simulink model "SPGF_FSK_0000_R2019b"  (R2019b)
settings: Solver=ode3  SolverName=ode4  StartTime=0.0  StopTime=1.4  FixedStep=50e-6/50  RelTol=1e-3  EnableMultiTasking=on
undefined symbols (not defined in the file): D11, Delta
libraries: powerlib x2544, powerlib_meascontrol x204, simulink x24
(part 20 of 33)

== system SPGF_FSK_0000_R2019b/W32/DPL ==
  Ccs2/1 : powerlib/Elements/Series RLC Branch  LConnTagsString=__new0  RConnTagsString=__new0  BranchType=R  Resistance=-Rg_matrix(3,4)*2  Inductance=1e-3  SetiL0=off  InitialCurrent=0  Capacitance=Rg_matrix(3,4)*2  Setx0=off  InitialVoltage=0  Measurements=None
  Ccs2/3 : powerlib/Elements/Series RLC Branch  LConnTagsString=__new0  RConnTagsString=__new0  BranchType=R  Resistance=-Rg_matrix(3,4)*2  Inductance=1e-3  SetiL0=off  InitialCurrent=0  Capacitance=Rg_matrix(3,4)*2  Setx0=off  InitialVoltage=0  Measurements=None
  Ccs3/1 : powerlib/Elements/Series RLC Branch  LConnTagsString=__new0  RConnTagsString=__new0  BranchType=R  Resistance=-Rg_matrix(5,6)*2  Inductance=1e-3  SetiL0=off  InitialCurrent=0  Capacitance=-C_matrix(5,6)/2  Setx0=off  InitialVoltage=0  Measurements=None
  Ccs3/3 : powerlib/Elements/Series RLC Branch  LConnTagsString=__new0  RConnTagsString=__new0  BranchType=R  Resistance=-Rg_matrix(5,6)*2  Inductance=1e-3  SetiL0=off  InitialCurrent=0  Capacitance=-C_matrix(5,6)/2  Setx0=off  InitialVoltage=0  Measurements=None
  DPL : powerlib/Elements/Distributed Parameters Line  Phases=6  Length=LineLength  Frequency=Frequency  Resistance=R_matrix  Inductance=L_matrix  Capacitance=C_matrix  x1=[-2.15e-05 -1.53014718047574 0 -11.9975076801494 0 0 -9002.7612999088;-2.1e-05 -1.53058650120651 0 -12.0009749818967 0 0 -9001.97102364387;-2.05e-05 -1.53102578417156 0 -12.0044419875317 0 0 -9001.18052526422;-2e-05 -1.53146502936007 0 -12.0079086969691 0 0 -9000.38980478933;-1.95e-05 -1.5319042367612 0 -12.0113751101231 0 0 -8999.59886223873;-1.9e-05 -1.5323434063641 0 -12.0148412269084 0 0 -8998.80769763193;-1.85e-05 -1.53278253815794 0 -12.0183070472393 0 0 -8998.01631098845;-1.8e-05 -1.53322163213189 0 -12.0217725710304 0 0 -8997.22470232782;-1.75e-05 -1.53366068827512 0 -12.0252377981962 0 0 -8996.43287166957;-1.7e-05 -1.53409970657678 0 -12.0287027286511 0 0 -8995.64081903323;-1.65e-05 -1.53453868702605 0 -12.0321673623096 0 0 -8994.84854443835;-1.6e-05 -1.5349776296121 0 -12.0356316990864 0 0 -8994.05604790448;-1.55e-05 -1.53541653432409 0 -12.0390957388958 0 0 -8993.26332945117;-1.5e-05 -1.53585540115119 0 -12.0425594816524 0 0 -8992.47038909799;-1.45e-05 -1.53629423008259 0 -12.0460229272708 0 0 -8991.67722686449;-1.4e-05 -1.53673302110744 0 -12.0494860756655 0 0 -8990.88384277025;-1.35e-05 -1.53717177421492 0 -12.052948926751 0 0 -8990.09023683485;-1.3e-05 -1.53761048939422 0 -12.056411480442 0 0 -8989.29640907786;-1.25e-05 -1.53804916663449 0 -12.0598737366529 0 0 -8988.50235951887;-1.2e-05 -1.53848780592492 0 -12.0633356952984 0 0 -8987.70808817747;-1.15e-05 -1.53892640725469 0 -12.066797356293 0 0 -8986.91359507327;-1.1e-05 -1.53936497061297 0 -12.0702587195513 0 0 -8986.11888022586;-1.05e-05 -1.53980349598894 0 -12.0737197849879 0 0 -8985.32394365486;-1e-05 -1.54024198337178 0 -12.0771805525174 0 0 -8984.52878537988;-9.5e-06 -1.54068043275068 0 -12.0806410220544 0 0 -8983.73340542053;-9e-06 -1.54111884411481 0 -12.0841011935135 0 0 -8982.93780379645;-8.5e-06 -1.54155721745336 0 -12.0875610668094 0 0 -8982.14198052726;-8e-06 -1.5419955527555 0 -12.0910206418567 0 0 -8981.3459356326;-7.5e-06 -1.54243385001044 0 -12.09447991857 0 0 -8980.54966913212;-7e-06 -1.54287210920734 0 -12.097938896864 0 0 -8979.75318104545;-6.5e-06 -1.5433103303354 0 -12.1013975766533 0 0 -8978.95647139226;-6e-06 -1.5437485133838 0 -12.1048559578526 0 0 -8978.15954019219;-5.5e-06 -1.54418665834174 0 -12.1083140403766 0 0 -8977.36238746492;-5e-06 -1.54462476519839 0 -12.1117718241398 0 0 -8976.56501323011;-4.5e-06 -1.54506283394296 0 -12.1152293090571 0 0 -8975.76741750744;-4e-06 -1.54550086456463 0 -12.1186864950431 -2674.88891077229 0 -8974.96960031658;-3.5e-06 -1.5459388570526 5072.52279858498 -12.1221433820125 -2675.63246615166 4735.28985862403 -8974.17156167723;-3e-06 -1.54637681139605 5073.93232204557 -12.12559996988 -2676.37595551245 4734.86865062958 -8973.37330160906;-2.5e-06 -1.54681472758419 5075.3417203119 -12.1290562585602 -2677.1193788363 4734.44732580693 -8972.57482013179;-2e-06 -1.5472526056062 5076.75099334919 -12.1325122479681 -2677.86273610488 4734.02588416648 -8971.77611726511;-1.5e-06 -1.54769044545128 5078.16014112268 -12.1359679380182 -2678.60602729985 4733.60432571862 -8970.97719302872;-1e-06 -1.54812824710863 5079.56916359758 -12.1394233286252 -2679.34925240286 4733.18265047376 -8970.17804744235;-5e-07 -1.54856601056745 5080.97806073914 -12.1428784197041 -2680.09241139558 4732.76085844229 -8969.3786805257]  x2=[-2.15e-05 -1.52937369923623 0 -11.9860465797701 0 0 -9022.25103677801;-2.1e-05 -1.52981566216544 0 -11.9895391205462 0 0 -9021.46040632605;-2.05e-05 -1.53025758734796 0 -11.9930313654924 0 0 -9020.66955327848;-2e-05 -1.5306994747729 0 -11.9965233145224 0 0 -9019.87847765481;-1.95e-05 -1.53114132442933 0 -12.00001496755 0 0 -9019.08717947456;-1.9e-05 -1.53158313630637 0 -12.0035063244892 0 0 -9018.29565875726;-1.85e-05 -1.53202491039311 0 -12.0069973852536 0 0 -9017.50391552242;-1.8e-05 -1.53246664667865 0 -12.0104881497573 0 0 -9016.7119497896;-1.75e-05 -1.53290834515209 0 -12.0139786179141 0 0 -9015.91976157833;-1.7e-05 -1.53335000580254 0 -12.0174687896379 0 0 -9015.12735090815;-1.65e-05 -1.53379162861909 0 -12.0209586648425 0 0 -9014.33471779863;-1.6e-05 -1.53423321359085 0 -12.0244482434418 0 0 -9013.54186226931;-1.55e-05 -1.53467476070692 0 -12.0279375253497 0 0 -9012.74878433976;-1.5e-05 -1.5351162699564 0 -12.0314265104802 0 0 -9011.95548402955;-1.45e-05 -1.53555774132842 0 -12.0349151987472 0 0 -9011.16196135825;-1.4e-05 -1.53599917481206 0 -12.0384035900645 0 0 -9010.36821634544;-1.35e-05 -1.53644057039645 0 -12.0418916843461 0 0 -9009.57424901071;-1.3e-05 -1.53688192807068 0 -12.0453794815059 0 0 -9008.78005937364;-1.25e-05 -1.53732324782387 0 -12.0488669814579 0 0 -9007.98564745383;-1.2e-05 -1.53776452964513 0 -12.0523541841161 0 0 -9007.19101327089;-1.15e-05 -1.53820577352357 0 -12.0558410893943 0 0 -9006.39615684442;-1.1e-05 -1.53864697944831 0 -12.0593276972066 0 0 -9005.60107819403;-1.05e-05 -1.53908814740845 0 -12.0628140074669 0 0 -9004.80577733934;-1e-05 -1.53952927739312 0 -12.0663000200891 0 0 -9004.01025429998;-9.5e-06 -1.53997036939142 0 -12.0697857349874 0 0 -9003.21450909557;-9e-06 -1.54041142339248 0 -12.0732711520756 0 0 -9002.41854174574;-8.5e-06 -1.54085243938541 0 -12.0767562712678 0 0 -9001.62235227014;-8e-06 -1.54129341735933 0 -12.080241092478 0 0 -9000.82594068841;-7.5e-06 -1.54173435730336 0 -12.0837256156202 0 0 -9000.02930702021;-7e-06 -1.54217525920661 0 -12.0872098406084 0 0 -8999.23245128518;-6.5e-06 -1.54261612305822 0 -12.0906937673567 0 0 -8998.43537350299;-6e-06 -1.5430569488473 0 -12.0941773957791 0 0 -8997.63807369331;-5.5e-06 -1.54349773656298 0 -12.0976607257895 0 0 -8996.84055187581;-5e-06 -1.54393848619438 0 -12.1011437573022 0 0 -8996.04280807017;-4.5e-06 -1.54437919773062 0 -12.1046264902311 0 0 -8995.24484229607;-4e-06 -1.54481987116083 0 -12.1081089244904 -2677.09103389761 0 -8994.4466545732;-3.5e-06 -1.54526050647415 5076.70076594894 -12.111591059994 -2677.83624236647 4745.56687862651 -8993.64824492125;-3e-06 -1.54570110365968 5078.11342326981 -12.1150728966561 -2678.58138476238 4745.14547461087 -8992.84961335993;-2.5e-06 -1.54614166270657 5079.52595529325 -12.1185544343908 -2679.32646106693 4744.72395351346 -8992.05075990894;-2e-06 -1.54658218360395 5080.93836198442 -12.1220356731121 -2680.07147126176 4744.30231534468 -8991.25168458799;-1.5e-06 -1.54702266634093 5082.35064330845 -12.1255166127341 -2680.81641532848 4743.88056011494 -8990.45238741679;-1e-06 -1.54746311090667 5083.76279923051 -12.1289972531711 -2681.5612932487 4743.45868783463 -8989.65286841508;-5e-07 -1.54790351729028 5085.17482971575 -12.132477594337 -2682.30610500404 4743.03669851417 -8988.85312760257]  x3=[-2.15e-05 0.00477826196837518 0 -0.618760489523996 0 0 -226.302645481419;-2.1e-05 0.00477462202162191 0 -0.619060199625067 0 0 -226.29417562915;-2.05e-05 0.00477098195705956 0 -0.619359894451439 0 0 -226.285700193296;-2e-05 0.00476734177477795 0 -0.619659573995719 0 0 -226.277219174067;-1.95e-05 0.00476370147486689 0 -0.619959238250512 0 0 -226.26873257167;-1.9e-05 0.00476006105741622 0 -0.620258887208423 0 0 -226.260240386317;-1.85e-05 0.00475642052251574 0 -0.62055852086206 0 0 -226.251742618216;-1.8e-05 0.00475277987025529 0 -0.620858139204029 0 0 -226.243239267577;-1.75e-05 0.0047491391007247 0 -0.621157742226938 0 0 -226.234730334609;-1.7e-05 0.0047454982140138 0 -0.621457329923394 0 0 -226.226215819524;-1.65e-05 0.00474185721021243 0 -0.621756902286004 0 0 -226.21769572253;-1.6e-05 0.00473821608941042 0 -0.622056459307379 0 0 -226.209170043839;-1.55e-05 0.00473457485169761 0 -0.622356000980125 0 0 -226.20063878366;-1.5e-05 0.00473093349716385 0 -0.622655527296852 0 0 -226.192101942204;-1.45e-05 0.00472729202589899 0 -0.622955038250171 0 0 -226.183559519681;-1.4e-05 0.00472365043799287 0 -0.623254533832689 0 0 -226.175011516303;-1.35e-05 0.00472000873353535 0 -0.623554014037019 0 0 -226.16645793228;-1.3e-05 0.00471636691261628 0 -0.62385347885577 0 0 -226.157898767824;-1.25e-05 0.00471272497532552 0 -0.624152928281553 0 0 -226.149334023145;-1.2e-05 0.00470908292175294 0 -0.62445236230698 0 0 -226.140763698455;-1.15e-05 0.00470544075198839 0 -0.624751780924663 0 0 -226.132187793965;-1.1e-05 0.00470179846612174 0 -0.625051184127214 0 0 -226.123606309887;-1.05e-05 0.00469815606424287 0 -0.625350571907245 0 0 -226.115019246433;-1e-05 0.00469451354644164 0 -0.625649944257368 0 0 -226.106426603814;-9.5e-06 0.00469087091280794 0 -0.625949301170199 0 0 -226.097828382243;-9e-06 0.00468722816343163 0 -0.626248642638349 0 0 -226.089224581932;-8.5e-06 0.00468358529840261 0 -0.626547968654434 0 0 -226.080615203092;-8e-06 0.00467994231781075 0 -0.626847279211067 0 0 -226.072000245937;-7.5e-06 0.00467629922174594 0 -0.627146574300863 0 0 -226.063379710679;-7e-06 0.00467265601029807 0 -0.627445853916438 0 0 -226.054753597531;-6.5e-06 0.00466901268355704 0 -0.627745118050407 0 0 -226.046121906705;-6e-06 0.00466536924161274 0 -0.628044366695387 0 0 -226.037484638415;-5.5e-06 0.00466172568455507 0 -0.628343599843992 0 0 -226.028841792873;-5e-06 0.00465808201247392 0 -0.628642817488841 0 0 -226.020193370294;-4.5e-06 0.00465443822545921 0 -0.62894201962255 0 0 -226.011539370889;-4e-06 0.00465079432360084 0 -0.629241206237737 -222.82339661273 0 -226.002879794873;-3.5e-06 0.00464715030698872 42.9134986181816 -0.629540377327019 -222.889214995494 448.335934563766 -225.99421464246;-3e-06 0.00464350617571277 42.9459643816412 -0.629839532883015 -222.955027878687 448.298611391661 -225.985543913863;-2.5e-06 0.00463986192986288 42.9784290854516 -0.630138672898344 -223.020835260686 448.261277158231 -225.976867609297;-2e-06 0.004636217569529 43.0108927288118 -0.630437797365624 -223.086637139865 448.223931864398 -225.968185728974;-1.5e-06 0.00463257309480103 43.0433553109208 -0.630736906277475 -223.152433514603 448.186575511082 -225.95949827311;-1e-06 0.00462892850576891 43.0758168309775 -0.631035999626517 -223.218224383275 448.149208099206 -225.950805241919;-5e-07 0.00462528380252255 43.1082772881811 -0.631335077405369 -223.284009744258 448.111829629691 -225.942106635616]  x4=[-2.15e-05 -0.0246566983072682 0 -0.809678743743674 0 0 -37.8270818179801;-2.1e-05 -0.0246588297990929 0 -0.809794272225366 0 0 -37.8124114690117;-2.05e-05 -0.0246609606824854 0 -0.809909780726186 0 0 -37.7977401870595;-2e-05 -0.0246630909573931 0 -0.810025269243283 0 0 -37.7830679724853;-1.95e-05 -0.0246652206237634 0 -0.810140737773807 0 0 -37.7683948256514;-1.9e-05 -0.0246673496815438 0 -0.81025618631491 0 0 -37.7537207469197;-1.85e-05 -0.0246694781306817 0 -0.810371614863743 0 0 -37.7390457366522;-1.8e-05 -0.0246716059711247 0 -0.810487023417458 0 0 -37.7243697952112;-1.75e-05 -0.0246737332028202 0 -0.810602411973208 0 0 -37.7096929229586;-1.7e-05 -0.0246758598257157 0 -0.810717780528144 0 0 -37.6950151202566;-1.65e-05 -0.0246779858397588 0 -0.810833129079422 0 0 -37.6803363874674;-1.6e-05 -0.024680111244897 0 -0.810948457624193 0 0 -37.6656567249532;-1.55e-05 -0.0246822360410779 0 -0.811063766159614 0 0 -37.6509761330762;-1.5e-05 -0.024684360228249 0 -0.811179054682838 0 0 -37.6362946121986;-1.45e-05 -0.0246864838063579 0 -0.811294323191021 0 0 -37.6216121626826;-1.4e-05 -0.0246886067753522 0 -0.81140957168132 0 0 -37.6069287848905;-1.35e-05 -0.0246907291351796 0 -0.811524800150889 0 0 -37.5922444791847;-1.3e-05 -0.0246928508857877 0 -0.811640008596887 0 0 -37.5775592459274;-1.25e-05 -0.0246949720271241 0 -0.811755197016471 0 0 -37.562873085481;-1.2e-05 -0.0246970925591365 0 -0.811870365406797 0 0 -37.5481859982079;-1.15e-05 -0.0246992124817726 0 -0.811985513765026 0 0 -37.5334979844704;-1.1e-05 -0.02470133179498 0 -0.812100642088315 0 0 -37.518809044631;-1.05e-05 -0.0247034504987065 0 -0.812215750373824 0 0 -37.5041191790521;-1e-05 -0.0247055685928998 0 -0.812330838618713 0 0 -37.4894283880961;-9.5e-06 -0.0247076860775076 0 -0.812445906820141 0 0 -37.4747366721256;-9e-06 -0.0247098029524777 0 -0.81256095497527 0 0 -37.460044031503;-8.5e-06 -0.0247119192177578 0 -0.812675983081262 0 0 -37.4453504665908;-8e-06 -0.0247140348732958 0 -0.812790991135277 0 0 -37.4306559777517;-7.5e-06 -0.0247161499190394 0 -0.812905979134479 0 0 -37.4159605653482;-7e-06 -0.0247182643549365 0 -0.813020947076029 0 0 -37.4012642297428;-6.5e-06 -0.0247203781809348 0 -0.813135894957092 0 0 -37.3865669712983;-6e-06 -0.0247224913969823 0 -0.813250822774831 0 0 -37.3718687903771;-5.5e-06 -0.0247246040030267 0 -0.81336573052641 0 0 -37.3571696873421;-5e-06 -0.024726715999016 0 -0.813480618208994 0 0 -37.3424696625559;-4.5e-06 -0.024728827384898 0 -0.813595485819749 0 0 -37.3277687163811;-4e-06 -0.0247309381606206 0 -0.813710333355839 -211.777509166727 0 -37.3130668491806;-3.5e-06 -0.0247330483261319 84.5050032625513 -0.813825160814432 -211.832740480619 382.91660687957 -37.2983640613171;-3e-06 -0.0247351578813796 84.5080140470438 -0.813939968192694 -211.887966567748 382.880140777377 -37.2836603531533;-2.5e-06 -0.0247372668263117 84.5110227463845 -0.814054755487792 -211.943187426751 382.843665227995 -37.268955725052;-2e-06 -0.0247393751608763 84.5140293604994 -0.814169522696895 -211.998403056265 382.807180232325 -37.2542501773762;-1.5e-06 -0.0247414828850213 84.5170338893141 -0.814284269817169 -212.053613454928 382.770685791266 -37.2395437104886;-1e-06 -0.0247435899986946 84.5200363327547 -0.814398996845785 -212.108818621378 382.734181905718 -37.224836324752;-5e-07 -0.0247456965018443 84.5230366907469 -0.814513703779911 -212.164018554253 382.697668576584 -37.2101280205295]  x5=2.11324941411031e-05  V1=ones(3,3)  V2=ones(3,3)  I1=ones(3,3)  I2=ones(3,3)  nHarmo=1  Measurements=None  Decoupling=off  VsMag0=0  VrMag0=0  VsAngle0=0  VrAngle0=0  IsMag0=0  IrMag0=0  IsAngle0=0  IrAngle0=0
  Ground{1..4} (4 alike) : powerlib/Elements/Ground  LConnTagsString=a
  Rcs*1 : powerlib/Elements/Series RLC Branch  LConnTagsString=__new0  RConnTagsString=__new0  BranchType=R  Resistance=-Rg_matrix(1,2)*2  Inductance=1e-3  SetiL0=off  InitialCurrent=0  Capacitance=Rg_matrix(1,2)*2  Setx0=off  InitialVoltage=0  Measurements=None
  Rcs*2 : powerlib/Elements/Series RLC Branch  LConnTagsString=__new0  RConnTagsString=__new0  BranchType=R  Resistance=-Rg_matrix(1,2)*2  Inductance=1e-3  SetiL0=off  InitialCurrent=0  Capacitance=Rg_matrix(1,2)*2  Setx0=off  InitialVoltage=0  Measurements=None
  Rgsg1/1 : powerlib/Elements/Series RLC Branch  LConnTagsString=__new0  RConnTagsString=__new0  BranchType=R  Resistance=(Rg_matrix(4,4)+Rg_matrix(3,4))*2  Inductance=1e-3  SetiL0=off  InitialCurrent=0  Capacitance=Rg_matrix(1,2)*2  Setx0=off  InitialVoltage=0  Measurements=None
  Rgsg1/2 : powerlib/Elements/Series RLC Branch  LConnTagsString=__new0  RConnTagsString=__new0  BranchType=R  Resistance=(Rg_matrix(2,2)+Rg_matrix(1,2))*2  Inductance=1e-3  SetiL0=off  InitialCurrent=0  Capacitance=Rg_matrix(1,2)*2  Setx0=off  InitialVoltage=0  Measurements=None
  Rgsg1/3 : powerlib/Elements/Series RLC Branch  LConnTagsString=__new0  RConnTagsString=__new0  BranchType=R  Resistance=(Rg_matrix(4,4)+Rg_matrix(3,4))*2  Inductance=1e-3  SetiL0=off  InitialCurrent=0  Capacitance=Rg_matrix(1,2)*2  Setx0=off  InitialVoltage=0  Measurements=None
  Rgsg1/4 : powerlib/Elements/Series RLC Branch  LConnTagsString=__new0  RConnTagsString=__new0  BranchType=R  Resistance=(Rg_matrix(2,2)+Rg_matrix(1,2))*2  Inductance=1e-3  SetiL0=off  InitialCurrent=0  Capacitance=Rg_matrix(1,2)*2  Setx0=off  InitialVoltage=0  Measurements=None
  Rsg*1 : powerlib/Elements/Series RLC Branch  LConnTagsString=__new0  RConnTagsString=__new0  BranchType=R  Resistance=(Rg_matrix(6,6)+Rg_matrix(5,6))*2  Inductance=1e-3  SetiL0=off  InitialCurrent=0  Capacitance=Rg_matrix(1,2)*2  Setx0=off  InitialVoltage=0  Measurements=None
  Rsg*2 : powerlib/Elements/Series RLC Branch  LConnTagsString=__new0  RConnTagsString=__new0  BranchType=R  Resistance=(Rg_matrix(6,6)+Rg_matrix(5,6))*2  Inductance=1e-3  SetiL0=off  InitialCurrent=0  Capacitance=Rg_matrix(1,2)*2  Setx0=off  InitialVoltage=0  Measurements=None
  A : PMIOPort  Side=Left
  B : PMIOPort  Port=2  Side=Left
  C : PMIOPort  Port=3  Side=Left
  a : PMIOPort  Port=4  Side=Right
  b : PMIOPort  Port=5  Side=Right
  c : PMIOPort  Port=6  Side=Right
  connections:
  c/RConn1 -- Ccs3/1/RConn1 -- DPL/RConn5
  b/RConn1 -- Ccs2/1/RConn1 -- DPL/RConn3
  a/RConn1 -- DPL/RConn1 -- Rcs*1/RConn1
  Ground4/LConn1 -- DPL/RConn6 -- Ccs3/1/LConn1 -- Rsg*1/LConn1 -- Rcs*1/LConn1 -- Rgsg1/4/LConn1 -- DPL/RConn2 -- DPL/RConn4 -- Ccs2/1/LConn1 -- Rgsg1/3/LConn1
  Ground1/LConn1 -- Rgsg1/4/RConn1 -- Rsg*1/RConn1 -- Rgsg1/3/RConn1
  Ground3/LConn1 -- Ccs3/3/LConn1 -- Rsg*2/LConn1 -- DPL/LConn6 -- Rgsg1/1/LConn1 -- Ccs2/3/LConn1 -- DPL/LConn4 -- Rgsg1/2/LConn1 -- Rcs*2/LConn1 -- DPL/LConn2
  Ground2/LConn1 -- Rgsg1/1/RConn1 -- Rsg*2/RConn1 -- Rgsg1/2/RConn1
  Ccs3/3/RConn1 -- DPL/LConn5 -- C/RConn1
  Ccs2/3/RConn1 -- DPL/LConn3 -- B/RConn1
  Rcs*2/RConn1 -- DPL/LConn1 -- A/RConn1

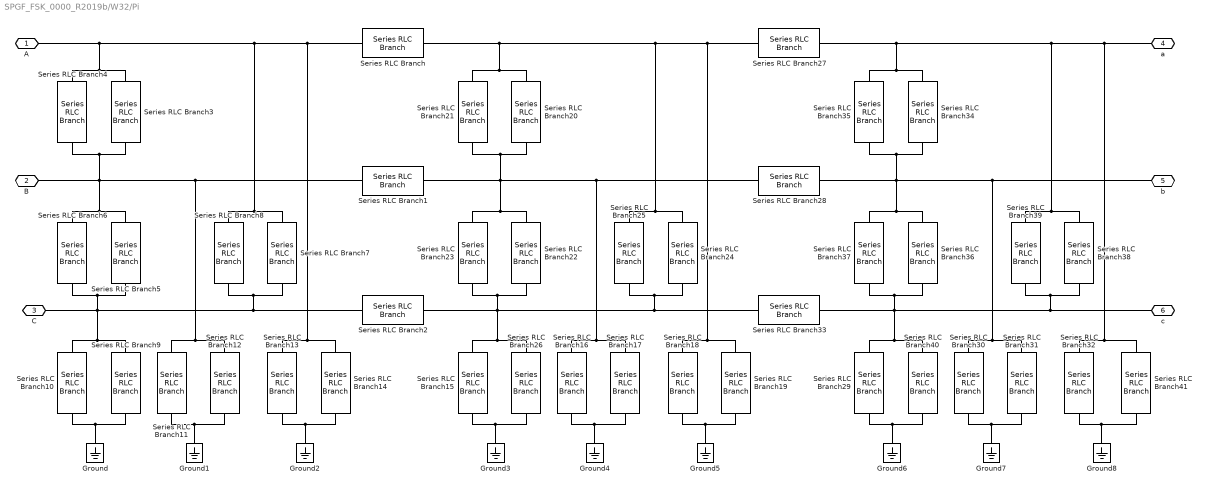
== system SPGF_FSK_0000_R2019b/W32/Pi ==
  Ground{,1..8} (9 alike) : powerlib/Elements/Ground  LConnTagsString=a
  Series RLC Branch{,1..2,27..28,33} (6 alike) : powerlib/Elements/Series RLC Branch  LConnTagsString=__new0  RConnTagsString=__new0  BranchType=RL  Resistance=R/2  Inductance=L/2  SetiL0=off  InitialCurrent=0  Capacitance=1e-6  Setx0=off  InitialVoltage=0  Measurements=None
  Series RLC Branch{10..11,13,29..30,32} (6 alike) : powerlib/Elements/Series RLC Branch  LConnTagsString=__new0  RConnTagsString=__new0  BranchType=R  Resistance=Rfg*4  Inductance=L/2  SetiL0=off  InitialCurrent=0  Capacitance=1e-6  Setx0=off  InitialVoltage=0  Measurements=None
  Series RLC Branch{9,12,14,31,40..41} (6 alike) : powerlib/Elements/Series RLC Branch  LConnTagsString=__new0  RConnTagsString=__new0  BranchType=C  Resistance=R/2  Inductance=L/2  SetiL0=off  InitialCurrent=0  Capacitance=Cfg*0.25  Setx0=off  InitialVoltage=0  Measurements=None
  Series RLC Branch15 : powerlib/Elements/Series RLC Branch  LConnTagsString=__new0  RConnTagsString=__new0  BranchType=R  Resistance=Rfg*2  Inductance=L/2  SetiL0=off  InitialCurrent=0  Capacitance=1e-6  Setx0=off  InitialVoltage=0  Measurements=None
  Series RLC Branch16 : powerlib/Elements/Series RLC Branch  LConnTagsString=__new0  RConnTagsString=__new0  BranchType=R  Resistance=Rfg*2  Inductance=L/2  SetiL0=off  InitialCurrent=0  Capacitance=1e-6  Setx0=off  InitialVoltage=0  Measurements=None
  Series RLC Branch17 : powerlib/Elements/Series RLC Branch  LConnTagsString=__new0  RConnTagsString=__new0  BranchType=C  Resistance=R/2  Inductance=L/2  SetiL0=off  InitialCurrent=0  Capacitance=Cfg*0.5  Setx0=off  InitialVoltage=0  Measurements=None
  Series RLC Branch18 : powerlib/Elements/Series RLC Branch  LConnTagsString=__new0  RConnTagsString=__new0  BranchType=R  Resistance=Rfg*2  Inductance=L/2  SetiL0=off  InitialCurrent=0  Capacitance=1e-6  Setx0=off  InitialVoltage=0  Measurements=None
  Series RLC Branch19 : powerlib/Elements/Series RLC Branch  LConnTagsString=__new0  RConnTagsString=__new0  BranchType=C  Resistance=R/2  Inductance=L/2  SetiL0=off  InitialCurrent=0  Capacitance=Cfg*0.5  Setx0=off  InitialVoltage=0  Measurements=None
  Series RLC Branch20 : powerlib/Elements/Series RLC Branch  LConnTagsString=__new0  RConnTagsString=__new0  BranchType=C  Resistance=R/2  Inductance=L/2  SetiL0=off  InitialCurrent=0  Capacitance=Cmf*0.5  Setx0=off  InitialVoltage=0  Measurements=None
  Series RLC Branch21 : powerlib/Elements/Series RLC Branch  LConnTagsString=__new0  RConnTagsString=__new0  BranchType=R  Resistance=Rmf*2  Inductance=L/2  SetiL0=off  InitialCurrent=0  Capacitance=1e-6  Setx0=off  InitialVoltage=0  Measurements=None
  Series RLC Branch22 : powerlib/Elements/Series RLC Branch  LConnTagsString=__new0  RConnTagsString=__new0  BranchType=C  Resistance=R/2  Inductance=L/2  SetiL0=off  InitialCurrent=0  Capacitance=Cmf*0.5  Setx0=off  InitialVoltage=0  Measurements=None
  Series RLC Branch23 : powerlib/Elements/Series RLC Branch  LConnTagsString=__new0  RConnTagsString=__new0  BranchType=R  Resistance=Rmf*2  Inductance=L/2  SetiL0=off  InitialCurrent=0  Capacitance=1e-6  Setx0=off  InitialVoltage=0  Measurements=None
  Series RLC Branch24 : powerlib/Elements/Series RLC Branch  LConnTagsString=__new0  RConnTagsString=__new0  BranchType=C  Resistance=R/2  Inductance=L/2  SetiL0=off  InitialCurrent=0  Capacitance=Cmf*0.5  Setx0=off  InitialVoltage=0  Measurements=None
  Series RLC Branch25 : powerlib/Elements/Series RLC Branch  LConnTagsString=__new0  RConnTagsString=__new0  BranchType=R  Resistance=Rmf*2  Inductance=L/2  SetiL0=off  InitialCurrent=0  Capacitance=1e-6  Setx0=off  InitialVoltage=0  Measurements=None
  Series RLC Branch26 : powerlib/Elements/Series RLC Branch  LConnTagsString=__new0  RConnTagsString=__new0  BranchType=C  Resistance=R/2  Inductance=L/2  SetiL0=off  InitialCurrent=0  Capacitance=Cfg*0.5  Setx0=off  InitialVoltage=0  Measurements=None
  Series RLC Branch{3,5,7,34,36,38} (6 alike) : powerlib/Elements/Series RLC Branch  LConnTagsString=__new0  RConnTagsString=__new0  BranchType=C  Resistance=R/2  Inductance=L/2  SetiL0=off  InitialCurrent=0  Capacitance=Cmf*0.25  Setx0=off  InitialVoltage=0  Measurements=None
  Series RLC Branch{4,6,8,35,37,39} (6 alike) : powerlib/Elements/Series RLC Branch  LConnTagsString=__new0  RConnTagsString=__new0  BranchType=R  Resistance=Rmf*4  Inductance=L/2  SetiL0=off  InitialCurrent=0  Capacitance=1e-6  Setx0=off  InitialVoltage=0  Measurements=None
  A : PMIOPort  Side=Left
  B : PMIOPort  Port=2  Side=Left
  C : PMIOPort  Port=3  Side=Left
  a : PMIOPort  Port=4  Side=Right
  b : PMIOPort  Port=5  Side=Right
  c : PMIOPort  Port=6  Side=Right
  connections:
  Ground8/LConn1 -- Series RLC Branch41/RConn1 -- Series RLC Branch32/RConn1
  Ground7/LConn1 -- Series RLC Branch30/RConn1 -- Series RLC Branch31/RConn1
  Ground6/LConn1 -- Series RLC Branch40/RConn1 -- Series RLC Branch29/RConn1
  Series RLC Branch40/LConn1 -- Series RLC Branch33/RConn1 -- Series RLC Branch38/RConn1 -- Series RLC Branch39/RConn1 -- c/RConn1 -- Series RLC Branch37/RConn1 -- Series RLC Branch36/RConn1 -- Series RLC Branch29/LConn1
  Series RLC Branch35/LConn1 -- Series RLC Branch27/RConn1 -- Series RLC Branch39/LConn1 -- Series RLC Branch38/LConn1 -- Series RLC Branch32/LConn1 -- Series RLC Branch41/LConn1 -- a/RConn1 -- Series RLC Branch34/LConn1
  Series RLC Branch30/LConn1 -- Series RLC Branch28/RConn1 -- Series RLC Branch37/LConn1 -- Series RLC Branch36/LConn1 -- Series RLC Branch34/RConn1 -- Series RLC Branch35/RConn1 -- b/RConn1 -- Series RLC Branch31/LConn1
  Series RLC Branch19/RConn1 -- Series RLC Branch18/RConn1 -- Ground5/LConn1
  Series RLC Branch16/RConn1 -- Series RLC Branch17/RConn1 -- Ground4/LConn1
  Ground3/LConn1 -- Series RLC Branch15/RConn1 -- Series RLC Branch26/RConn1
  Series RLC Branch23/RConn1 -- Series RLC Branch22/RConn1 -- Series RLC Branch24/RConn1 -- Series RLC Branch25/RConn1 -- Series RLC Branch33/LConn1 -- Series RLC Branch2/RConn1 -- Series RLC Branch15/LConn1 -- Series RLC Branch26/LConn1
  Series RLC Branch25/LConn1 -- Series RLC Branch24/LConn1 -- Series RLC Branch18/LConn1 -- Series RLC Branch19/LConn1 -- Series RLC Branch27/LConn1 -- Series RLC Branch/RConn1 -- Series RLC Branch20/LConn1 -- Series RLC Branch21/LConn1
  Series RLC Branch21/RConn1 -- Series RLC Branch20/RConn1 -- Series RLC Branch22/LConn1 -- Series RLC Branch23/LConn1 -- Series RLC Branch1/RConn1 -- Series RLC Branch28/LConn1 -- Series RLC Branch16/LConn1 -- Series RLC Branch17/LConn1
  Ground2/LConn1 -- Series RLC Branch14/RConn1 -- Series RLC Branch13/RConn1
  Ground1/LConn1 -- Series RLC Branch11/RConn1 -- Series RLC Branch12/RConn1
  Series RLC Branch10/RConn1 -- Ground/LConn1 -- Series RLC Branch9/RConn1
  Series RLC Branch10/LConn1 -- Series RLC Branch6/RConn1 -- Series RLC Branch5/RConn1 -- C/RConn1 -- Series RLC Branch7/RConn1 -- Series RLC Branch8/RConn1 -- Series RLC Branch2/LConn1 -- Series RLC Branch9/LConn1
  Series RLC Branch14/LConn1 -- Series RLC Branch/LConn1 -- Series RLC Branch8/LConn1 -- Series RLC Branch7/LConn1 -- Series RLC Branch3/LConn1 -- Series RLC Branch4/LConn1 -- A/RConn1 -- Series RLC Branch13/LConn1
  Series RLC Branch1/LConn1 -- Series RLC Branch3/RConn1 -- Series RLC Branch4/RConn1 -- B/RConn1 -- Series RLC Branch6/LConn1 -- Series RLC Branch5/LConn1 -- Series RLC Branch11/LConn1 -- Series RLC Branch12/LConn1

== system SPGF_FSK_0000_R2019b/W32/Q ==
  breaker : Subsystem  Commented=on  mask{SwitchA=off, SwitchB=off, SwitchC=off, InitialStatus=[1 1 1], BreakerResistance=0.0001, SnubberResistance=1e6, SnubberCapacitance=inf, TransitionTimes=[0.5 0.7], ShiftTimes=[0 0 0]}
      mask prompts: SwitchA "Switching of phase A"; SwitchB "Switching of phase B"; SwitchC "Switching of phase C"; InitialStatus "Initial status of phase breaker [A, B, C]"; BreakerResistance "Breaker resistance Ron (ohms) :"; SnubberResistance "Snubbers resistance Rp (ohms) :"; SnubberCapacitance "Snubbers capacitance Cp (F) :"; TransitionTimes "Transition times (s) :"; ShiftTimes "Time differences for switch [tA, tB, tC] (s) :"
      mask init: same as SPGF_FSK_0000_R2019b/Feed/Q/breaker
      mask Display:
      | % port_label('input',1,'Iabc');
      | 
      | port_label('lconn',1,'A');
      | port_label('lconn',2,'B');
      | port_label('lconn',3,'C');
      | 
      | port_label('rconn',1,'a');
      | port_label('rconn',2,'b');
      | port_label('rconn',3,'c');
      | 
      | disp('   Q    ');
  meas : Subsystem
  shunt : Subsystem
  A : PMIOPort  Side=Right
  B : PMIOPort  Port=2  Side=Right
  C : PMIOPort  Port=3  Side=Right
  a : PMIOPort  Port=4  Side=Left
  b : PMIOPort  Port=5  Side=Left
  c : PMIOPort  Port=6  Side=Left
  connections:
  shunt/LConn3 -- C/RConn1 -- breaker/LConn3
  shunt/LConn2 -- B/RConn1 -- breaker/LConn2
  A/RConn1 -- shunt/LConn1 -- breaker/LConn1
  meas/RConn1 -- a/RConn1
  meas/RConn2 -- b/RConn1
  meas/RConn3 -- c/RConn1
  meas/LConn3 -- breaker/RConn3 -- shunt/RConn3
  meas/LConn2 -- breaker/RConn2 -- shunt/RConn2
  meas/LConn1 -- breaker/RConn1 -- shunt/RConn1

== system SPGF_FSK_0000_R2019b/W32/concentrated ==
  Ccs/1 : powerlib/Elements/Series RLC Branch  LConnTagsString=__new0  RConnTagsString=__new0  BranchType=C  Resistance=190  Inductance=1e-3  SetiL0=off  InitialCurrent=0  Capacitance=-C_matrix(1,2)/2  Setx0=off  InitialVoltage=0  Measurements=None
  Ccs/2 : powerlib/Elements/Series RLC Branch  LConnTagsString=__new0  RConnTagsString=__new0  BranchType=C  Resistance=190  Inductance=1e-3  SetiL0=off  InitialCurrent=0  Capacitance=-C_matrix(1,2)/2  Setx0=off  InitialVoltage=0  Measurements=None
  Ccs2/1 : powerlib/Elements/Series RLC Branch  LConnTagsString=__new0  RConnTagsString=__new0  BranchType=C  Resistance=190  Inductance=1e-3  SetiL0=off  InitialCurrent=0  Capacitance=-C_matrix(3,4)/2  Setx0=off  InitialVoltage=0  Measurements=None
  Ccs2/2 : powerlib/Elements/Series RLC Branch  LConnTagsString=__new0  RConnTagsString=__new0  BranchType=C  Resistance=190  Inductance=1e-3  SetiL0=off  InitialCurrent=0  Capacitance=-C_matrix(3,4)/2  Setx0=off  InitialVoltage=0  Measurements=None
  Ccs2/3 : powerlib/Elements/Series RLC Branch  LConnTagsString=__new0  RConnTagsString=__new0  BranchType=R  Resistance=-Rg_matrix(3,4)*2  Inductance=1e-3  SetiL0=off  InitialCurrent=0  Capacitance=Rg_matrix(3,4)*2  Setx0=off  InitialVoltage=0  Measurements=None
  Ccs2/4 : powerlib/Elements/Series RLC Branch  LConnTagsString=__new0  RConnTagsString=__new0  BranchType=R  Resistance=-Rg_matrix(3,4)*2  Inductance=1e-3  SetiL0=off  InitialCurrent=0  Capacitance=Rg_matrix(3,4)*2  Setx0=off  InitialVoltage=0  Measurements=None
  Ccs3/1 : powerlib/Elements/Series RLC Branch  LConnTagsString=__new0  RConnTagsString=__new0  BranchType=C  Resistance=190  Inductance=1e-3  SetiL0=off  InitialCurrent=0  Capacitance=-C_matrix(5,6)/2  Setx0=off  InitialVoltage=0  Measurements=None
  Ccs3/2 : powerlib/Elements/Series RLC Branch  LConnTagsString=__new0  RConnTagsString=__new0  BranchType=C  Resistance=190  Inductance=1e-3  SetiL0=off  InitialCurrent=0  Capacitance=-C_matrix(5,6)/2  Setx0=off  InitialVoltage=0  Measurements=None
  Ccs3/3 : powerlib/Elements/Series RLC Branch  LConnTagsString=__new0  RConnTagsString=__new0  BranchType=R  Resistance=-Rg_matrix(5,6)*2  Inductance=1e-3  SetiL0=off  InitialCurrent=0  Capacitance=-C_matrix(5,6)/2  Setx0=off  InitialVoltage=0  Measurements=None
  Ccs3/4 : powerlib/Elements/Series RLC Branch  LConnTagsString=__new0  RConnTagsString=__new0  BranchType=R  Resistance=-Rg_matrix(5,6)*2  Inductance=1e-3  SetiL0=off  InitialCurrent=0  Capacitance=-C_matrix(5,6)/2  Setx0=off  InitialVoltage=0  Measurements=None
  Csg/2 : powerlib/Elements/Series RLC Branch  LConnTagsString=__new0  RConnTagsString=__new0  BranchType=C  Resistance=190  Inductance=1e-3  SetiL0=off  InitialCurrent=0  Capacitance=( C_matrix(1,2) + C_matrix(2,2) )/2  Setx0=off  InitialVoltage=0  Measurements=None
  Csg1/1 : powerlib/Elements/Series RLC Branch  LConnTagsString=__new0  RConnTagsString=__new0  BranchType=C  Resistance=190  Inductance=1e-3  SetiL0=off  InitialCurrent=0  Capacitance=( C_matrix(1,2) + C_matrix(2,2) )/2  Setx0=off  InitialVoltage=0  Measurements=None
  Csg2/1 : powerlib/Elements/Series RLC Branch  LConnTagsString=__new0  RConnTagsString=__new0  BranchType=C  Resistance=190  Inductance=1e-3  SetiL0=off  InitialCurrent=0  Capacitance=( C_matrix(3,4) + C_matrix(4,4) )/2  Setx0=off  InitialVoltage=0  Measurements=None
  Csg2/2 : powerlib/Elements/Series RLC Branch  LConnTagsString=__new0  RConnTagsString=__new0  BranchType=C  Resistance=190  Inductance=1e-3  SetiL0=off  InitialCurrent=0  Capacitance=( C_matrix(3,4) + C_matrix(4,4) )/2  Setx0=off  InitialVoltage=0  Measurements=None
  Csg3/1 : powerlib/Elements/Series RLC Branch  LConnTagsString=__new0  RConnTagsString=__new0  BranchType=C  Resistance=190  Inductance=1e-3  SetiL0=off  InitialCurrent=0  Capacitance=( C_matrix(5,6) + C_matrix(6,6) ) /2  Setx0=off  InitialVoltage=0  Measurements=None
  Csg3/2 : powerlib/Elements/Series RLC Branch  LConnTagsString=__new0  RConnTagsString=__new0  BranchType=C  Resistance=190  Inductance=1e-3  SetiL0=off  InitialCurrent=0  Capacitance=( C_matrix(5,6) + C_matrix(6,6) ) /2  Setx0=off  InitialVoltage=0  Measurements=None
  Ground{1..4} (4 alike) : powerlib/Elements/Ground  LConnTagsString=a
  RL : powerlib/Elements/Mutual Inductance  LConnTagsString=a|b|c|L4|L5|L6  RConnTagsString=A|B|C|R4|R5|R6  TypeOfMutual=Generalized mutual inductance  NumberOfWindings=6  SelfImpedance1=[1.1 1.1e-03]  SelfImpedance2=[ 1.1 1.1e-03]  ThreeWindings=on  SelfImpedance3=[ 1.1 1.1e-03]  MutualImpedance=[1.0 1.0e-03]  InductanceMatrix=L_matrix  ResistanceMatrix=R_matrix  Measurements=None
      settings: AttributesFormatString=\n
  Rcs*2 : powerlib/Elements/Series RLC Branch  LConnTagsString=__new0  RConnTagsString=__new0  BranchType=R  Resistance=-Rg_matrix(1,2)*2  Inductance=1e-3  SetiL0=off  InitialCurrent=0  Capacitance=Rg_matrix(1,2)*2  Setx0=off  InitialVoltage=0  Measurements=None
  Rgcs1/1 : powerlib/Elements/Series RLC Branch  LConnTagsString=__new0  RConnTagsString=__new0  BranchType=R  Resistance=-Rg_matrix(1,2)*2  Inductance=1e-3  SetiL0=off  InitialCurrent=0  Capacitance=Rg_matrix(1,2)*2  Setx0=off  InitialVoltage=0  Measurements=None
  Rgsg1/1 : powerlib/Elements/Series RLC Branch  LConnTagsString=__new0  RConnTagsString=__new0  BranchType=R  Resistance=(Rg_matrix(4,4)+Rg_matrix(3,4))*2  Inductance=1e-3  SetiL0=off  InitialCurrent=0  Capacitance=Rg_matrix(1,2)*2  Setx0=off  InitialVoltage=0  Measurements=None
  Rgsg1/2 : powerlib/Elements/Series RLC Branch  LConnTagsString=__new0  RConnTagsString=__new0  BranchType=R  Resistance=(Rg_matrix(2,2)+Rg_matrix(1,2))*2  Inductance=1e-3  SetiL0=off  InitialCurrent=0  Capacitance=Rg_matrix(1,2)*2  Setx0=off  InitialVoltage=0  Measurements=None
  Rgsg1/3 : powerlib/Elements/Series RLC Branch  LConnTagsString=__new0  RConnTagsString=__new0  BranchType=R  Resistance=(Rg_matrix(4,4)+Rg_matrix(3,4))*2  Inductance=1e-3  SetiL0=off  InitialCurrent=0  Capacitance=Rg_matrix(1,2)*2  Setx0=off  InitialVoltage=0  Measurements=None
  Rgsg1/4 : powerlib/Elements/Series RLC Branch  LConnTagsString=__new0  RConnTagsString=__new0  BranchType=R  Resistance=(Rg_matrix(2,2)+Rg_matrix(1,2))*2  Inductance=1e-3  SetiL0=off  InitialCurrent=0  Capacitance=Rg_matrix(1,2)*2  Setx0=off  InitialVoltage=0  Measurements=None
  Rsg*2 : powerlib/Elements/Series RLC Branch  LConnTagsString=__new0  RConnTagsString=__new0  BranchType=R  Resistance=(Rg_matrix(6,6)+Rg_matrix(5,6))*2  Inductance=1e-3  SetiL0=off  InitialCurrent=0  Capacitance=Rg_matrix(1,2)*2  Setx0=off  InitialVoltage=0  Measurements=None
  Rsg1/1 : powerlib/Elements/Series RLC Branch  LConnTagsString=__new0  RConnTagsString=__new0  BranchType=R  Resistance=(Rg_matrix(6,6)+Rg_matrix(5,6))*2  Inductance=1e-3  SetiL0=off  InitialCurrent=0  Capacitance=Rg_matrix(1,2)*2  Setx0=off  InitialVoltage=0  Measurements=None
  A : PMIOPort  Side=Left
  B : PMIOPort  Port=2  Side=Left
  C : PMIOPort  Port=3  Side=Left
  a : PMIOPort  Port=4  Side=Right
  b : PMIOPort  Port=5  Side=Right
  c : PMIOPort  Port=6  Side=Right
  connections:
  Ccs3/3/RConn1 -- RL/LConn5 -- C/RConn1 -- Ccs3/2/RConn1
  Ccs2/2/RConn1 -- Ccs2/3/RConn1 -- B/RConn1 -- RL/LConn3
  Ccs/2/RConn1 -- Rcs*2/RConn1 -- A/RConn1 -- RL/LConn1
  Ccs3/4/RConn1 -- RL/RConn5 -- c/RConn1 -- Ccs3/1/RConn1
  Ccs2/1/RConn1 -- Ccs2/4/RConn1 -- RL/RConn3 -- b/RConn1
  Ccs/1/RConn1 -- Rgcs1/1/RConn1 -- RL/RConn1 -- a/RConn1
  Csg/2/RConn1 -- Ground1/LConn1 -- Csg2/2/RConn1 -- Csg3/2/RConn1 -- Rgsg1/2/RConn1 -- Rgsg1/1/RConn1 -- Rsg*2/RConn1
  Csg3/1/LConn1 -- Ccs3/4/LConn1 -- Rsg1/1/LConn1 -- Ccs3/1/LConn1 -- RL/RConn6 -- Ground4/LConn1 -- RL/RConn2 -- Ccs/1/LConn1 -- Csg1/1/LConn1 -- Rgcs1/1/LConn1 -- Rgsg1/4/LConn1 -- RL/RConn4 -- Ccs2/1/LConn1 -- Csg2/1/LConn1 -- Ccs2/4/LConn1 -- Rgsg1/3/LConn1
  Csg1/1/RConn1 -- Ground2/LConn1 -- Csg2/1/RConn1 -- Csg3/1/RConn1 -- Rgsg1/4/RConn1 -- Rgsg1/3/RConn1 -- Rsg1/1/RConn1
  Ccs3/2/LConn1 -- Ccs3/3/LConn1 -- Csg3/2/LConn1 -- Rsg*2/LConn1 -- Ccs2/2/LConn1 -- Ccs2/3/LConn1 -- Csg2/2/LConn1 -- Rgsg1/1/LConn1 -- RL/LConn4 -- RL/LConn2 -- Ccs/2/LConn1 -- Rcs*2/LConn1 -- Csg/2/LConn1 -- Rgsg1/2/LConn1 -- Ground3/LConn1 -- RL/LConn6
